simulink model "AWES3_CL_wTether_v4_PM"  (R2022a)
settings: Solver=ode3  StartTime=0  StopTime=simInit.TSIM  FixedStep=simInit.dt  RelTol=1e-3
values from neighbouring files (symbols this model uses):
  complex_tether_flag = 1    [run_sim.m]
  Ft_max = 1870    [run_sim.m]
  q = 0    [barrier_optimization.m]
  r = 0    [barrier_optimization.m]
  random_seed = [ 24335       17059       17670        1747]    [run_sim.m]
  safety_controller = false    [run_sim.m]
  turbulence = true    [run_sim.m]
undefined symbols (not defined in the file or in its folder): aeroModel, alpha_max, alpha_min, alpha_options, base_windspeed, constr, DiscIntNeverNeededParam, dx, ENVMT, F, grid_max, grid_min, HDBK, I_table, Light, MIL, mu_max, mu_min, mu_options, P_AP2, params, SampleTime, simInit, T, u0_sim, winchParameter, x0_sim
libraries: simulink x30, aerolibwind2 x14, dspstat3 x2, pid_lib x1, aerolibwindfilters x1, aerolibcommonsys x1, matrix_library x1
(part 3 of 5)

== system AWES3_CL_wTether_v4_PM/FlightController/Retraction/CalculateAttitudeCmds ==
  pathangles_k_cmd : Inport
  Ft_set : Inport  Port=2
  F_t_m : Inport  Port=3
  airdata : Inport  Port=4
  v_w_O : Inport  Port=5
  v_k_O : Inport  Port=6
  p_G_O : Inport  Port=7
  pathangles_a : Inport  Port=8
  mu_a : Inport  Port=9
  Demux{1..4} (4 alike) : Demux  Outputs=2
  Dot Product : DotProduct  OutDataTypeStr=Inherit: Inherit via internal rule
  FlightPathLoopRetraction : Subsystem
  FlightpathReferenceModels : Subsystem
  Gain : Gain  Gain=0.5*1.225
  Mux1 : Mux  Commented=on  Inputs=3
  Mux3 : Mux  Commented=on  Inputs=3
  PIController_opt : Subsystem
  Product : Product
  Saturation : Saturate  UpperLimit=constr.alpha_a_max  LowerLimit=constr.alpha_a_min
  Scope1 : Scope  Commented=on
  Scope2 : Scope  Commented=on
  Selector : Selector  InputPortWidth=3  IndexOptions=Index vector (dialog)  Indices=1  OutputSizes=1
  Selector1 : Selector  InputPortWidth=3  IndexOptions=Index vector (dialog)  Indices=3  OutputSizes=1
  Sqrt : Sqrt
  Sum : Sum  Inputs=|+-
  Sum1 : Sum  Inputs=|+-
  Terminator : Terminator
  Terminator1 : Terminator
  TrafoPathKin2PathAero : MATLAB Function  TreatAsAtomicUnit=on
  mu_a_cmd : Outport  VectorParamsAs1DForOutWhenUnconnected=off
  alpha_cmd : Outport  Port=2  VectorParamsAs1DForOutWhenUnconnected=off
  wires:
  FlightPathLoopRetraction/1(mu_a_c) -> mu_a_cmd/1
  pathangles_a/1 -> FlightPathLoopRetraction/5(pathangles_a), Demux4/1, PIController_opt/3(path_angles_a)
  p_G_O/1 -> FlightPathLoopRetraction/6(p_G_O)
  FlightPathLoopRetraction/3(Ft) -> Terminator1/1
  FlightPathLoopRetraction/4(push_mode) -> Terminator/1
  FlightPathLoopRetraction/6(gamma_dot_real) -> Sum1/2
  pathangles_k_cmd/1 -> Demux2/1
  Ft_set/1 -> FlightPathLoopRetraction/2(F_t_set)
  Selector1/1 -> TrafoPathKin2PathAero/6(beta)
  TrafoPathKin2PathAero/2(gamma_a) -> FlightpathReferenceModels/2(gamma_cmd), Mux3/1
  TrafoPathKin2PathAero/1(chi_a) -> FlightpathReferenceModels/1(chi_cmd), Mux1/1
  Selector/1 -> TrafoPathKin2PathAero/2(Va), Product/1, Product/2  "Va"
  Sqrt/1 -> TrafoPathKin2PathAero/1(Vg)
  Dot Product/1 -> Sqrt/1
  FlightPathLoopRetraction/2(alpha_a_c) -> Saturation/1
  PIController_opt/1(nu_a_path) -> Demux1/1, FlightPathLoopRetraction/3(nu_a_path)
  Sum1/1 -> FlightpathReferenceModels/4(gamma_hedge)
  FlightPathLoopRetraction/5(chi_dot_real) -> Sum/2
  Demux1/2 -> Sum1/1
  Demux1/1 -> Sum/1
  FlightpathReferenceModels/1(xD_ref) -> PIController_opt/1(dot_Ref)
  Demux2/1 -> TrafoPathKin2PathAero/4(chi_k)
  FlightpathReferenceModels/2(x_ref) -> Demux3/1, PIController_opt/2(x_ref)
  Demux2/2 -> TrafoPathKin2PathAero/3(gamma_k)
  Demux3/1 -> Mux1/2
  Demux4/2 -> Mux3/3
  Demux3/2 -> Mux3/2
  Demux4/1 -> Mux1/3
  Product/1 -> Gain/1
  Gain/1 -> FlightpathReferenceModels/5(dynamic_pressure)
  Mux1/1 -> Scope1/1
  Mux3/1 -> Scope2/1
  Sum/1 -> FlightpathReferenceModels/3(chi_hedge)
  F_t_m/1 -> FlightPathLoopRetraction/1(F_t_m)
  airdata/1 -> FlightPathLoopRetraction/4(airdata), Selector1/1, Selector/1
  v_w_O/1 -> TrafoPathKin2PathAero/5(v_w_O)
  v_k_O/1 -> Dot Product/2, Dot Product/1
  mu_a/1 -> FlightPathLoopRetraction/7(mu_a)
  Saturation/1 -> alpha_cmd/1

== system AWES3_CL_wTether_v4_PM/FlightController/Retraction/GuidanceFlatEarth ==
  pos_G_O : Inport
  "vel_K_O " : Inport  Port=2
  phi0_retraction : Inport  Port=3
  Va : Inport  Port=4
  Chart : Stateflow chart  TreatAsAtomicUnit=on  mask{vamin_max=params.vamin_max, vamin=params.vamin, vamax=params.vamax, vamax_min=params.vamax_min}
  Constant : Constant  Value=params.vamin_max
  Delay1 : Delay  DelayLength=1  InitialConditionSource=Input port  InitialCondition=zeros(3,1)
      settings: InputPortMap=u0,p4
  Delay2 : Delay  DelayLength=1
  Dot Product3 : DotProduct  OutDataTypeStr=Inherit: Inherit via internal rule
  Gain1 : Gain  Gain=params.KpVaControl
  Gain3 : Gain  Gain=-1
  Gain5 : Gain  Gain=-1
  MATLAB Function1 : MATLAB Function  TreatAsAtomicUnit=on
  Mux : Mux  Inputs=2
  Mux1 : Mux  Inputs=2
  Saturation1 : Saturate  UpperLimit=constr.gamma_retraction_max  LowerLimit=constr.gamma_retraction_min
  Sqrt1 : Sqrt
  Sum : Sum  Inputs=|+-
  Sum1 : Sum  Inputs=++|
  Switch : Switch  Criteria=u2 > Threshold  SaturateOnIntegerOverflow=off  InputSameDT=off
  Terminator1 : Terminator
  calculateTransitionTrigger1 : MATLAB Function  TreatAsAtomicUnit=on
  d2r : Gain  Gain=pi/180
  approachFlag : Outport  VectorParamsAs1DForOutWhenUnconnected=off
  course_path : Outport  Port=2  VectorParamsAs1DForOutWhenUnconnected=off
  transition_flag : Outport  Port=3  VectorParamsAs1DForOutWhenUnconnected=off
  flag_pos_W : Outport  Port=4  VectorParamsAs1DForOutWhenUnconnected=off
  retraction_path_error : Outport  Port=5  VectorParamsAs1DForOutWhenUnconnected=off
  target_W : Outport  Port=6  VectorParamsAs1DForOutWhenUnconnected=off
  wires:
  Mux/1 -> course_path/1
  calculateTransitionTrigger1/2(transition_flag) -> transition_flag/1
  calculateTransitionTrigger1/7(flag_pos_y_W) -> flag_pos_W/1
  pos_G_O/1 -> Gain3/1, calculateTransitionTrigger1/2(pos_G_O_m)
  Delay1/1 -> Gain5/1, Delay1/1
  "vel_K_O "/1 -> Dot Product3/1, Dot Product3/2, MATLAB Function1/1(vel_k_O)
  Gain3/1 -> Delay1/2
  Dot Product3/1 -> Sqrt1/1
  Sqrt1/1 -> calculateTransitionTrigger1/4(v_k_tot)
  Gain5/1 -> calculateTransitionTrigger1/1(pos_init_retraction_O)
  calculateTransitionTrigger1/3(chi_k_cmd) -> Mux/1
  MATLAB Function1/2(vel_k_h_W) -> calculateTransitionTrigger1/3(vk_xy)
  MATLAB Function1/1(vel_k_down_W) -> Terminator1/1
  Saturation1/1 -> Mux/2  "gamma"
  calculateTransitionTrigger1/4(d_horizontal) -> Mux1/1
  calculateTransitionTrigger1/5(d_vertical) -> Mux1/2
  phi0_retraction/1 -> calculateTransitionTrigger1/5(phi0_retraction)
  calculateTransitionTrigger1/8(approachFlag) -> Delay2/1  "approachFlag"
  Delay2/1 -> approachFlag/1
  Chart/1(speed_by_pitch) -> Switch/2
  Switch/1 -> Saturation1/1
  Sum/1 -> Gain1/1
  Constant/1 -> Sum/2
  Va/1 -> calculateTransitionTrigger1/6(Va), Sum/1, Chart/2(va)  "va"
  Sum1/1 -> Switch/1
  d2r/1 -> Sum1/2
  calculateTransitionTrigger1/6(gamma_k_cmd) -> Sum1/1, Switch/3
  Gain1/1 -> d2r/1
  calculateTransitionTrigger1/9(flare_flag) -> Chart/1(flare_flag)  "flare_flag"
  Mux1/1 -> retraction_path_error/1
  calculateTransitionTrigger1/1(target_W) -> target_W/1

== system AWES3_CL_wTether_v4_PM/FlightController/Traction/FlightPathLoopTraction ==
  Ft_set : Inport
  F_a_B_est : Inport  Port=2  PortDimensions=[3,1]
  nu_chi : Inport  Port=3
  nu_gamma : Inport  Port=4
  pos_G_O : Inport  Port=5  PortDimensions=[3,1]
  airdata : Inport  Port=6  PortDimensions=[3,1]
  pathangles_k : Inport  Port=7  PortDimensions=[2,1]
  pathangles_a : Inport  Port=8  PortDimensions=[2,1]
  v_k_B : Inport  Port=9  PortDimensions=[3,1]
  mu_a_cmd : Inport  Port=10
  Constant : Constant  Value=0
  Delay{,2..5} (5 alike) : Delay  DelayLength=1  ExternalReset=Falling
      settings: InputPortMap=u0,r5
  Delay1 : Delay  DelayLength=1  InitialConditionSource=Input port  ExternalReset=Falling
      settings: InputPortMap=u0,r5,p4
  Demux : Demux  Outputs=2
  Demux1 : Demux  Outputs=2
  Demux2 : Demux  Outputs=2
  EstimatePlantResponse : Subsystem
  MATLAB Function : MATLAB Function  TreatAsAtomicUnit=on
  Mux : Mux  Inputs=2
  Saturation : Saturate  UpperLimit=constr.alpha_a_max  LowerLimit=constr.alpha_a_min
  Sum{,1..3} (4 alike) : Sum  Inputs=|+-
  inversionPathDynamics : MATLAB Function  TreatAsAtomicUnit=on
  inversionPathDynamics1 : MATLAB Function  Commented=on  TreatAsAtomicUnit=on
  mu_a_c_traction : Outport  PortDimensions=1  VectorParamsAs1DForOutWhenUnconnected=off
  alpha_rq : Outport  Port=2  PortDimensions=1  VectorParamsAs1DForOutWhenUnconnected=off
  wires:
  F_a_B_est/1 -> inversionPathDynamics/4(F_a_B_est)
  Demux1/1 -> inversionPathDynamics/6(chi_k)
  pathangles_a/1 -> inversionPathDynamics/9(pathangles_a)
  inversionPathDynamics/1(mu_a) -> mu_a_c_traction/1
  Mux/1 -> Demux/1
  Demux/2 -> inversionPathDynamics/3(nu_gamma_k)
  Demux/1 -> inversionPathDynamics/2(nu_chi_k)
  inversionPathDynamics/2(mu_k_c) -> EstimatePlantResponse/1(mu_k_sat)
  inversionPathDynamics/3(alpha_rq) -> Saturation/1
  inversionPathDynamics/4(dphi) -> EstimatePlantResponse/2(dphi)
  Delay1/1 -> inversionPathDynamics/11(L_rq_old)
  Delay/1 -> inversionPathDynamics/12(mu_a_old)
  MATLAB Function/1(L_rq) -> Delay1/3
  inversionPathDynamics/5(L_rq) -> Delay1/1
  Demux1/2 -> inversionPathDynamics/7(gamma_k)
  airdata/1 -> EstimatePlantResponse/8(airdata), inversionPathDynamics/10(airdata), MATLAB Function/1(airdata)
  pathangles_k/1 -> EstimatePlantResponse/5(chi_gamma_k), Demux1/1
  v_k_B/1 -> EstimatePlantResponse/7(v_k_B), inversionPathDynamics/8(v_k_B)
  pos_G_O/1 -> inversionPathDynamics/5(pos_O), EstimatePlantResponse/6(pos_O)
  Ft_set/1 -> EstimatePlantResponse/3(Ft), inversionPathDynamics/1(Ft_set)
  Delay5/1 -> Sum3/1
  nu_chi/1 -> Sum/1
  Sum3/1 -> Sum/2
  Delay4/1 -> Sum2/2
  Delay3/1 -> Sum3/2
  Demux2/2 -> Delay4/1
  Sum1/1 -> Delay2/1, Mux/2
  Sum/1 -> Delay5/1, Mux/1
  Delay2/1 -> Sum2/1
  EstimatePlantResponse/1(pathAngleRate) -> Demux2/1
  nu_gamma/1 -> Sum1/1
  Demux2/1 -> Delay3/1
  Sum2/1 -> Sum1/2
  mu_a_cmd/1 -> Delay/1
  Constant/1 -> Delay/2, Delay1/2, Delay2/2, Delay5/2, Delay4/2, Delay3/2
  Saturation/1 -> EstimatePlantResponse/4(alpha_rq), alpha_rq/1

== system AWES3_CL_wTether_v4_PM/FlightController/Traction/Ft_set_smoothing ==
  F_t_m : Inport
  Data Type Conversion : DataTypeConversion  OutDataTypeStr=boolean  SaturateOnIntegerOverflow=off  RndMeth=Floor
  force switch1 : Subsystem  Commented=on
  force switch2 : Subsystem
  recommend_switch : Outport
  Ft_set_out : Outport  Port=2
  wires:
  F_t_m/1 -> force switch2/1(u), Ft_set_out/1
  force switch2/1(Out) -> Data Type Conversion/1
  Data Type Conversion/1 -> recommend_switch/1

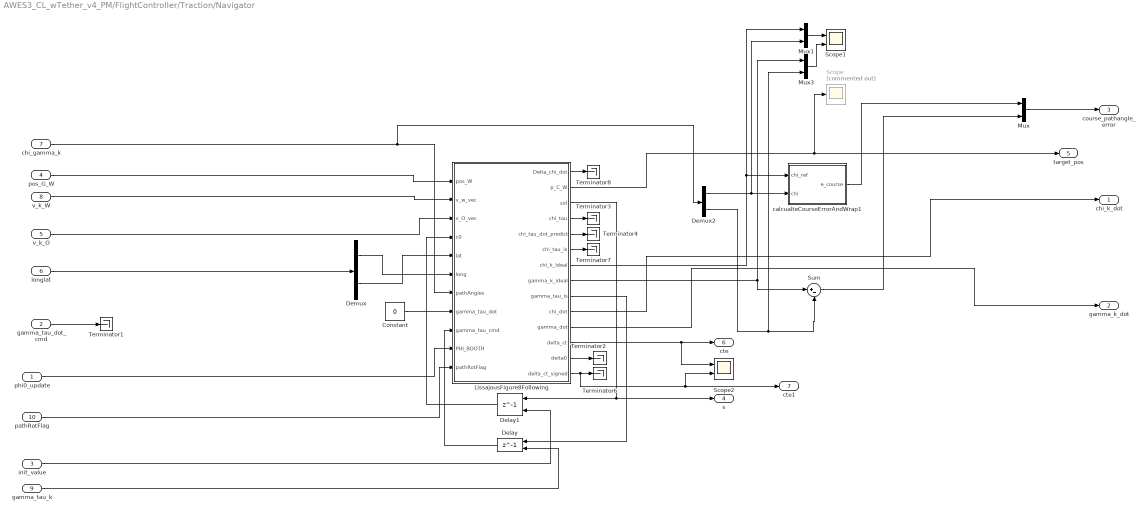
== system AWES3_CL_wTether_v4_PM/FlightController/Traction/Navigator ==
  phi0_update : Inport
  gamma_tau_dot_cmd : Inport  Port=2
  init_value : Inport  Port=3
  pos_G_W : Inport  Port=4
  v_k_O : Inport  Port=5
  longlat : Inport  Port=6  PortDimensions=2
  chi_gamma_k : Inport  Port=7
  v_k_W : Inport  Port=8
  gamma_tau_k : Inport  Port=9
  pathRotFlag : Inport  Port=10
  Constant : Constant  Value=0
  Delay : Delay  DelayLength=1  InitialConditionSource=Input port  InitialCondition=0
      settings: InputPortMap=u0,p4
  Delay1 : Delay  DelayLength=1  InitialConditionSource=Input port  InitialCondition=pi/2
      settings: InputPortMap=u0,p4
  Demux : Demux  Outputs=2
  Demux2 : Demux  Outputs=2
  LissajousFigure8Following : MATLAB Function  TreatAsAtomicUnit=on
  Mux : Mux  Inputs=2
  Mux1 : Mux  Inputs=2
  Mux3 : Mux  Inputs=2
  Scope : Scope  Commented=on
  Scope1 : Scope  NumInputPorts=2
  Scope2 : Scope  NumInputPorts=2
  Sum : Sum  Inputs=|+-
  Terminator{1..4,6..8} (7 alike) : Terminator
  calcualteCourseErrorAndWrap1 : MATLAB Function  TreatAsAtomicUnit=on
  chi_k_dot : Outport  PortDimensions=1  VectorParamsAs1DForOutWhenUnconnected=off
  gamma_k_dot : Outport  Port=2  PortDimensions=1  VectorParamsAs1DForOutWhenUnconnected=off
  "course_pathangle_error " : Outport  Port=3  VectorParamsAs1DForOutWhenUnconnected=off
  s : Outport  Port=4  PortDimensions=1  VectorParamsAs1DForOutWhenUnconnected=off
  target_pos : Outport  Port=5  VectorParamsAs1DForOutWhenUnconnected=off
  cte : Outport  Port=6  PortDimensions=1  VectorParamsAs1DForOutWhenUnconnected=off
  cte1 : Outport  Port=7  PortDimensions=1  VectorParamsAs1DForOutWhenUnconnected=off
  wires:
  Mux3/1 -> Scope1/2
  Mux1/1 -> Scope1/1
  LissajousFigure8Following/2(p_C_W) -> target_pos/1, Scope/1
  Delay1/1 -> LissajousFigure8Following/4(c0)
  LissajousFigure8Following/3(sol) -> Delay1/1, s/1
  v_k_O/1 -> LissajousFigure8Following/3(v_O_vec)
  Demux/1 -> LissajousFigure8Following/6(long)
  calcualteCourseErrorAndWrap1/1(e_course) -> Mux/1
  LissajousFigure8Following/7(chi_k_ideal) -> calcualteCourseErrorAndWrap1/1(chi_ref), Mux1/1
  Demux2/1 -> calcualteCourseErrorAndWrap1/2(chi), Mux1/2
  Demux2/2 -> Mux3/2, Sum/2
  Mux/1 -> "course_pathangle_error "/1
  LissajousFigure8Following/11(gamma_dot) -> gamma_k_dot/1
  LissajousFigure8Following/10(chi_dot) -> chi_k_dot/1
  Sum/1 -> Mux/2
  Demux/2 -> LissajousFigure8Following/5(lat)
  LissajousFigure8Following/9(gamma_tau_is) -> Delay/1
  pos_G_W/1 -> LissajousFigure8Following/1(pos_W)
  longlat/1 -> Demux/1
  chi_gamma_k/1 -> LissajousFigure8Following/7(pathAngles), Demux2/1
  gamma_tau_dot_cmd/1 -> Terminator1/1
  init_value/1 -> Delay1/2
  Constant/1 -> LissajousFigure8Following/8(gamma_tau_dot)
  v_k_W/1 -> LissajousFigure8Following/2(v_w_vec)
  LissajousFigure8Following/13(delta0) -> Terminator2/1
  LissajousFigure8Following/4(chi_tau) -> Terminator3/1
  LissajousFigure8Following/12(delta_ct) -> Scope2/1, cte/1
  LissajousFigure8Following/14(delta_ct_signed) -> Scope2/2, cte1/1, Terminator6/1
  LissajousFigure8Following/6(chi_tau_is) -> Terminator7/1
  LissajousFigure8Following/8(gamma_k_ideal) -> Mux3/1, Sum/1
  phi0_update/1 -> LissajousFigure8Following/10(PHI_BOOTH)
  LissajousFigure8Following/5(chi_tau_dot_predict) -> Terminator4/1
  gamma_tau_k/1 -> Delay/2
  pathRotFlag/1 -> LissajousFigure8Following/11(pathRotFlag)
  LissajousFigure8Following/1(Delta_chi_dot) -> Terminator8/1
  Delay/1 -> LissajousFigure8Following/9(gamma_tau_cmd)

== system AWES3_CL_wTether_v4_PM/FlightController/Traction/PI_controller_course ==
  In1 : Inport
  Demux : Demux  Outputs=2
  PI_controller_course_chi : Subsystem
  PI_controller_course_gamma : Subsystem
  chi_error : Outport
  gamma_error : Outport  Port=2
  wires:
  PI_controller_course_chi/1(u_PI_fb) -> chi_error/1  "chi_error"
  In1/1 -> Demux/1
  Demux/1 -> PI_controller_course_chi/1(e_chi)
  PI_controller_course_gamma/1(u_PI_fb) -> gamma_error/1  "gamma_error"
  Demux/2 -> PI_controller_course_gamma/1(e_gamma)

== system AWES3_CL_wTether_v4_PM/FlightController/Traction/Subsystem ==
  alpha_safety_cmd : Inport
  safety_switch : Inport  Port=2
  alpha_NDI_cmd : Inport  Port=3
  Gain4 : Gain
  Integrator3 : Integrator  ExternalReset=rising  InitialConditionSource=external
  Sum5 : Sum  Inputs=|+-
  Switch3 : Switch  Criteria=u2 > Threshold  SaturateOnIntegerOverflow=off  InputSameDT=off
  alpha_cmd : Outport
  wires:
  alpha_safety_cmd/1 -> Switch3/1, Sum5/1
  Gain4/1 -> Integrator3/1
  Sum5/1 -> Gain4/1
  safety_switch/1 -> Switch3/2, Integrator3/2
  Switch3/1 -> alpha_cmd/1  "alpha_cmd"
  Integrator3/1 -> Sum5/2  "alpha_safety_smooth"
  alpha_NDI_cmd/1 -> Integrator3/3, Switch3/3

== system AWES3_CL_wTether_v4_PM/FlightController/Traction/Subsystem1 ==
  mu_safety_cmd : Inport
  safety_switch : Inport  Port=2
  mu_NDI_cmd : Inport  Port=3
  Gain3 : Gain
  Integrator1 : Integrator  ExternalReset=rising  InitialConditionSource=external
  Sum3 : Sum  Inputs=|+-
  Switch2 : Switch  Criteria=u2 > Threshold  SaturateOnIntegerOverflow=off  InputSameDT=off
  mu_cmd : Outport
  wires:
  safety_switch/1 -> Switch2/2, Integrator1/2
  Switch2/1 -> mu_cmd/1  "mu_cmd"
  Gain3/1 -> Integrator1/1
  Sum3/1 -> Gain3/1
  mu_NDI_cmd/1 -> Integrator1/3, Switch2/3
  Integrator1/1 -> Sum3/2  "mu_safety_smooth"
  mu_safety_cmd/1 -> Switch2/1, Sum3/1

== system AWES3_CL_wTether_v4_PM/FlightController/Traction/Subsystem2 ==
  alpha_safety_cmd : Inport
  safety_switch : Inport  Port=2
  alpha_NDI_cmd : Inport  Port=3
  Gain4 : Gain  Gain=params.w0_mu_a_emulation
  Integrator3 : Integrator  ExternalReset=rising  InitialConditionSource=external
  Sum5 : Sum  Inputs=|+-
  Switch3 : Switch  Criteria=u2 > Threshold  SaturateOnIntegerOverflow=off  InputSameDT=off
  alpha_cmd : Outport
  wires:
  alpha_safety_cmd/1 -> Sum5/1
  Gain4/1 -> Integrator3/1
  Sum5/1 -> Gain4/1
  alpha_NDI_cmd/1 -> Integrator3/3, Switch3/3
  safety_switch/1 -> Switch3/2, Integrator3/2
  Switch3/1 -> alpha_cmd/1  "alpha_cmd"
  Integrator3/1 -> Sum5/2, Switch3/1  "alpha_safety_smooth"

== system AWES3_CL_wTether_v4_PM/FlightController/Traction/Subsystem3 ==
  s : Inport
  sigma : Inport  Port=2
  recommend_switch : Inport  Port=3
  h_tau : Inport  Port=4
  Va : Inport  Port=5
  chi_a : Inport  Port=6
  gamma_a : Inport  Port=7
  tether_diff : Inport  Port=8
  Enable : EnablePort  StatesWhenEnabling=reset
  Max : MinMax  Inputs=2
  Safety control : MATLAB Function  TreatAsAtomicUnit=on
  Saturation : Saturate  UpperLimit=constr.alpha_a_max  LowerLimit=constr.alpha_a_min
  safety_switch : Outport
  mu_safety_cmd : Outport  Port=2
  alpha_safety_cmd : Outport  Port=3
  in_BRS : Outport  Port=4
  wires:
  Safety control/2(mu_a) -> mu_safety_cmd/1  "mu_safety_cmd"
  sigma/1 -> Safety control/2(sigma)
  h_tau/1 -> Safety control/3(h_tau)
  Max/1 -> safety_switch/1  "safety_switch"
  Va/1 -> Safety control/4(Va)
  gamma_a/1 -> Safety control/6(gamma_a)
  tether_diff/1 -> Safety control/7(tether_diff)
  s/1 -> Safety control/1(s)
  chi_a/1 -> Safety control/5(chi_a)
  Safety control/3(alpha_a) -> Saturation/1  "alpha_safety_cmd"
  Safety control/1(value) -> in_BRS/1, Max/1  "in_BRS"
  recommend_switch/1 -> Max/2
  Saturation/1 -> alpha_safety_cmd/1

== system AWES3_CL_wTether_v4_PM/FlightController/Traction/alpha_actuator_delay1 ==
  alpha_cmd : Inport
  Gain : Gain  Gain=params.w0_alpha_a_emulation
  Integrator : Integrator  InitialConditionSource=external
  Sum2 : Sum  Inputs=|+-
  alpha_is : Outport
  wires:
  Integrator/1 -> Sum2/2, alpha_is/1
  Gain/1 -> Integrator/1
  alpha_cmd/1 -> Integrator/2, Sum2/1
  Sum2/1 -> Gain/1

== system AWES3_CL_wTether_v4_PM/FlightController/Traction/mu_actuator_delay ==
  mu_cmd : Inport
  Gain : Gain  Gain=params.w0_mu_a_emulation
  Integrator : Integrator  InitialConditionSource=external
  Sum2 : Sum  Inputs=|+-
  mu_is : Outport
  wires:
  Integrator/1 -> Sum2/2, mu_is/1  "mu_is"
  Gain/1 -> Integrator/1
  mu_cmd/1 -> Integrator/2, Sum2/1
  Sum2/1 -> Gain/1

== system AWES3_CL_wTether_v4_PM/Aircraft_Winch_Tether/Subsystem/6DoFKinematics1/LowPassFilter ==
  In1 : Inport
  Gain : Gain  Gain=w0
  Integrator : Integrator  InitialCondition=x0
  Sum2 : Sum  Inputs=|+-
  Out1 : Outport  VectorParamsAs1DForOutWhenUnconnected=off
  wires:
  Gain/1 -> Integrator/1
  Sum2/1 -> Gain/1
  In1/1 -> Sum2/1
  Integrator/1 -> Out1/1, Sum2/2

== system AWES3_CL_wTether_v4_PM/Aircraft_Winch_Tether/WinchDynamicsAndControl /PureTorqueControl/PI-ForceController ==
  preSat : Inport
  retraction : Inport  Port=2
  controlDeficitDue2Sat : Inport  Port=3
  e_Ft : Inport  Port=4
  Constant : Constant  Value=base_windspeed
  Constant1 : Constant  Value=9
  Constant3 : Constant  Value=7
  Constant4 : Constant
  Discrete-Time Integrator1 : DiscreteIntegrator  ExternalReset=either  SampleTime=-1  UpperSaturationLimit=winchParameter.omega_max  LowerSaturationLimit=winchParameter.omega_min  ICPrevOutput=DiscIntNeverNeededParam  ICPrevScaledInput=DiscIntNeverNeededParam
  Divide : Product  Inputs=*/
  Gain1 : Gain  Gain=2
  Gain2 : Gain  Gain=2
  Gain3 : Gain  Gain=60
  Gain8 : Gain  Gain=params.ki_winch
  Gain9 : Gain  Gain=params.kp_winch
  HighWindGain1 : Gain  Gain=0.5
  LowWindGain1 : Gain  Gain=0.5
  Product1 : Product
  Saturation Dynamic : simulink/Discontinuities/Saturation Dynamic  OutMin=[]  OutMax=[]  OutDataTypeStr=Inherit: Same as second input  OutDataType=fixdt(1, 16)  OutScaling=2^-10  DoSatur=off
  Sum : Sum  Inputs=|+-
  Sum1 : Sum  Inputs=|+-
  Sum2 : Sum  Inputs=|++
  Sum3 : Sum  Inputs=|-+
  Sum8 : Sum
  clamping_logic : Subsystem
  TorqueCmd : Outport  VectorParamsAs1DForOutWhenUnconnected=off
  wires:
  Gain9/1 -> Gain2/1
  Gain8/1 -> Gain1/1
  clamping_logic/1(pre_integration_processed) -> Discrete-Time Integrator1/1
  Gain1/1 -> clamping_logic/2(preInt)
  Discrete-Time Integrator1/1 -> Sum8/1
  Sum8/1 -> TorqueCmd/1
  e_Ft/1 -> Gain9/1, Gain8/1
  retraction/1 -> Discrete-Time Integrator1/2
  Constant/1 -> Saturation Dynamic/2
  Constant3/1 -> Sum1/2, Sum/2, Saturation Dynamic/3
  Saturation Dynamic/1 -> Sum/1
  Divide/1 -> HighWindGain1/1, Sum3/1
  HighWindGain1/1 -> Sum2/1
  Constant4/1 -> Sum3/2
  Sum3/1 -> LowWindGain1/1
  LowWindGain1/1 -> Sum2/2
  Product1/1 -> Sum8/2
  Sum2/1 -> Product1/2
  Constant1/1 -> Saturation Dynamic/1, Sum1/1
  Sum/1 -> Divide/1
  Sum1/1 -> Divide/2
  controlDeficitDue2Sat/1 -> clamping_logic/3(control_def)
  preSat/1 -> clamping_logic/1(preSat)
  Gain2/1 -> Product1/1

== system AWES3_CL_wTether_v4_PM/Aircraft_Winch_Tether/WinchDynamicsAndControl /PureTorqueControl/Subsystem ==
  In1 : Inport
  Gain1 : Gain  Gain=params.winch_control_filter_w0*0.25
  Integrator : Integrator
  Sum1 : Sum  Inputs=|+-
  Out1 : Outport  VectorParamsAs1DForOutWhenUnconnected=off
  wires:
  Sum1/1 -> Gain1/1
  Integrator/1 -> Out1/1, Sum1/2  "F_t_m"
  Gain1/1 -> Integrator/1
  In1/1 -> Sum1/1

== system AWES3_CL_wTether_v4_PM/Aircraft_Winch_Tether/WinchDynamicsAndControl /PureTorqueControl1/PI-ForceController ==
  RetractionFlag : Inport
  controlDeficitDue2Sat : Inport  Port=2
  e_Ft : Inport  Port=3
  Abs : Abs  SaturateOnIntegerOverflow=off
  Compare To Constant : simulink/Logic and Bit Operations/Compare To Constant  relop=>=  const=1e-3  OutDataTypeStr=boolean
  Constant2 : Constant  Value=0
  Discrete-Time Integrator1 : DiscreteIntegrator  ExternalReset=rising  SampleTime=simInit.dt  UpperSaturationLimit=winchParameter.omega_max  LowerSaturationLimit=winchParameter.omega_min  ICPrevOutput=DiscIntNeverNeededParam  ICPrevScaledInput=DiscIntNeverNeededParam
  Gain11 : Gain  Gain=0.5
  Gain7 : Gain  Gain=0.14
  Gain8 : Gain  Gain=params.ki_winch
  Gain9 : Gain  Gain=params.kp_winch
  Logical Operator : Logic  Operator=OR  AllPortsSameDT=off  OutDataTypeStr=boolean
  Scope : Scope
  Sum8 : Sum
  Switch : Switch  Criteria=u2 > Threshold  SaturateOnIntegerOverflow=off  InputSameDT=off
  TorqueCmd : Outport  VectorParamsAs1DForOutWhenUnconnected=off
  wires:
  ? -> Discrete-Time Integrator1/2
  RetractionFlag/1 -> Logical Operator/1
  e_Ft/1 -> Gain8/1, Gain9/1
  controlDeficitDue2Sat/1 -> Abs/1
  Sum8/1 -> TorqueCmd/1
  Abs/1 -> Compare To Constant/1
  Discrete-Time Integrator1/1 -> Sum8/1, Scope/1
  Compare To Constant/1 -> Logical Operator/2
  Gain11/1 -> Switch/3
  Switch/1 -> Discrete-Time Integrator1/1
  Gain8/1 -> Gain11/1
  Logical Operator/1 -> Switch/2
  Gain7/1 -> Sum8/2
  Gain9/1 -> Gain7/1
  Constant2/1 -> Switch/1

== system AWES3_CL_wTether_v4_PM/Aircraft_Winch_Tether/WinchDynamicsAndControl /PureTorqueControl2/PI-ForceController ==
  retraction : Inport
  controlDeficitDue2Sat : Inport  Port=2
  e_Ft : Inport  Port=3
  Abs : Abs  SaturateOnIntegerOverflow=off
  Compare To Constant : simulink/Logic and Bit Operations/Compare To Constant  relop=>  const=0  OutDataTypeStr=boolean
  Compare To Constant1 : simulink/Logic and Bit Operations/Compare To Constant  relop=<  const=0  OutDataTypeStr=boolean
  Constant : Constant  Value=base_windspeed
  Constant1 : Constant  Value=9
  Constant2 : Constant  Value=0
  Constant3 : Constant  Value=7
  Constant4 : Constant
  Discrete-Time Integrator1 : DiscreteIntegrator  ExternalReset=either  SampleTime=-1  UpperSaturationLimit=winchParameter.omega_max  LowerSaturationLimit=winchParameter.omega_min  ICPrevOutput=DiscIntNeverNeededParam  ICPrevScaledInput=DiscIntNeverNeededParam
  Divide : Product  Inputs=*/
  Gain1 : Gain  Gain=0.5
  Gain8 : Gain  Gain=params.ki_winch
  Gain9 : Gain  Gain=params.kp_winch
  HighWindGain : Gain  Gain=0.5
  Logical Operator : Logic  AllPortsSameDT=off  OutDataTypeStr=boolean
  LowWindGain : Gain  Gain=0.4
  PID Controller : pid_lib/PID Controller  Controller=PID  Form=Parallel  TimeDomain=Continuous-time  UseExternalTs=off  SampleTime=-1  IntegratorMethod=Forward Euler  FilterMethod=Forward Euler  ControllerParametersSource=internal  P=1  I=1  D=0  UseFilter=on  N=100  TunerSelectOption=Transfer Function Based (PID Tuner App)  InitialConditionSource=internal  InitialConditionForIntegrator=0  InitialConditionForFilter=0  DifferentiatorICPrevScaledInput=0  ExternalReset=none  TrackingMode=off  Kt=1  LimitOutput=on  SatLimitsSource=internal  UpperSaturationLimit=inf  LowerSaturationLimit=-inf  LinearizeAsGain=on  AntiWindupMode=clamping  Kb=1  POutMin=[]  POutMax=[]  IOutMin=[]  IOutMax=[]  DOutMin=[]  DOutMax=[]  NOutMin=[]  NOutMax=[]  SumOutMin=[]  SumOutMax=[]  SaturationOutMin=[]  SaturationOutMax=[]  PParamMin=[]  PParamMax=[]  IParamMin=[]  IParamMax=[]  DParamMin=[]  DParamMax=[]  NParamMin=[]  NParamMax=[]  KbParamMin=[]  KbParamMax=[]  KtParamMin=[]  KtParamMax=[]  KbOutMin=[]  KbOutMax=[]  KtOutMin=[]  KtOutMax=[]  IntegratorOutMin=[]  IntegratorOutMax=[]  FilterOutMin=[]  FilterOutMax=[]  SumI1OutMin=[]  SumI1OutMax=[]  SumI2OutMin=[]  SumI2OutMax=[]  SumI3OutMin=[]  SumI3OutMax=[]  SumI4OutMin=[]  SumI4OutMax=[]  SumDOutMin=[]  SumDOutMax=[]  DifferentiatorOutMin=[]  DifferentiatorOutMax=[]  FilterDiffOutCoefMin=[]  FilterDiffOutCoefMax=[]  ReciprocalOutMin=[]  ReciprocalOutMax=[]  SumDenOutMin=[]  SumDenOutMax=[]  SumNumOutMin=[]  SumNumOutMax=[]  DivideOutMin=[]  DivideOutMax=[]  UdiffTsProdOutMin=[]  UdiffTsProdOutMax=[]  NTsProdOutMin=[]  NTsProdOutMax=[]  UintegralTsProdOutMin=[]  UintegralTsProdOutMax=[]  UngainTsProdOutMin=[]  UngainTsProdOutMax=[]  IntegratorContinuousStateAttributes=''  IntegratorStateMustResolveToSignalObject=off  IntegratorRTWStateStorageClass=Auto  FilterContinuousStateAttributes=''  FilterStateMustResolveToSignalObject=off  FilterRTWStateStorageClass=Auto  ParallelPVariant=InternalParameters  IdealPVariant=Disabled  IVariant=InternalParameters  DVariant=InternalParameters  IntegratorVariant=Continuous  SatVariant=Enabled  AWVariant=ContClampingParallel  PCopyVariant=Disabled  TRVariant=Disabled  FdbkBlocksVariant=Forward  IdealPFdbkVariant=Disabled  SatFdbkVariant=Disabled  DerivativeFilterVariant=ContFilter  NVariant=InternalParameters  NCopyVariant=Disabled  FilterICVariant=InternalICsFilter  IntegratorICVariant=InternalICs  ExternalResetVariant=Disabled  TRSumVariant=Passthrough  SumFdbkVariant=Disabled  SumVariant=Sum_PID  TsampFilterVariant=InternalTs  TsampNgainVariant=Passthrough  TsampIntegralVariant=Passthrough  ExternalSaturationOutDataTypeStr=Inherit: Same as second input
  Product : Product
  Product1 : Product
  Saturation Dynamic : simulink/Discontinuities/Saturation Dynamic  OutMin=[]  OutMax=[]  OutDataTypeStr=Inherit: Same as second input  OutDataType=fixdt(1, 16)  OutScaling=2^-10  DoSatur=off
  Scope : Scope
  Sign : Signum
  Sign1 : Signum
  Sum : Sum  Inputs=|+-
  Sum1 : Sum  Inputs=|+-
  Sum2 : Sum  Inputs=|++
  Sum3 : Sum  Inputs=|-+
  Sum8 : Sum
  Switch : Switch  Criteria=u2 > Threshold  SaturateOnIntegerOverflow=off  InputSameDT=off
  TorqueCmd : Outport  VectorParamsAs1DForOutWhenUnconnected=off
  wires:
  Sum1/1 -> Divide/2
  Sum/1 -> Divide/1
  Constant1/1 -> Sum1/1, Saturation Dynamic/1
  Sum2/1 -> Product1/2
  Product1/1 -> Sum8/2
  LowWindGain/1 -> Sum2/2
  Sum3/1 -> LowWindGain/1
  Constant4/1 -> Sum3/2
  HighWindGain/1 -> Sum2/1
  Divide/1 -> HighWindGain/1, Sum3/1
  Saturation Dynamic/1 -> Sum/1
  Constant3/1 -> Saturation Dynamic/3, Sum/2, Sum1/2
  Constant/1 -> Saturation Dynamic/2
  retraction/1 -> Discrete-Time Integrator1/2
  Logical Operator/1 -> Switch/2
  Compare To Constant1/1 -> Logical Operator/1
  Product/1 -> Compare To Constant1/1
  Sign/1 -> Product/2
  Sign1/1 -> Product/1
  e_Ft/1 -> Gain8/1, Gain9/1, Sign1/1
  controlDeficitDue2Sat/1 -> Abs/1, Sign/1
  Sum8/1 -> TorqueCmd/1
  Abs/1 -> Compare To Constant/1
  Discrete-Time Integrator1/1 -> Sum8/1, Scope/1
  Compare To Constant/1 -> Logical Operator/2
  Gain1/1 -> Switch/3
  Switch/1 -> Discrete-Time Integrator1/1
  Gain8/1 -> Gain1/1
  Gain9/1 -> Product1/1
  Constant2/1 -> Switch/1

== system AWES3_CL_wTether_v4_PM/Aircraft_Winch_Tether/WindfieldModel/Subsystem1/Subsystem ==
  Altitude : Inport  Unit=m
  Airspeed : Inport  Port=2  Unit=m/s
  DCM : Inport  Port=3  Unit=1  PortDimensions=[3 3]
  (u,v,w) : Selector  InputPortWidth=4  IndexOptions=Index vector (dialog)  Indices=[1 2 3]  OutputSizes=1
  Angle Conversion : aerolibwind2/Dryden Wind Turbulence Model  (Continuous (+q -r))/Angle Conversion  SystemSampleTime=-1  VariantActivationTime=update diagram  Latency=0  AutoFrameSizeCalculation=off
      settings: SourceProductBaseCode=AE
  Bus Creator : BusCreator  Inputs=3
  Disallow CGS : UnitConfiguration  UnitSystemsStr=English,SI,SI (extended)  AllowAllUnitSystems=off
  Filters on angular rates : aerolibwind2/Dryden Wind Turbulence Model  (Continuous (+q -r))/Filters on angular rates  SystemSampleTime=-1  VariantActivationTime=update diagram  Latency=0  AutoFrameSizeCalculation=off
      settings: SourceProductBaseCode=AE
  Filters on velocities : aerolibwindfilters/Dryden Continuous Filters  SystemSampleTime=-1  VariantActivationTime=update diagram  Latency=0  AutoFrameSizeCalculation=off
      settings: SourceProductBaseCode=AE
  Length Conversion : aerolibwind2/Dryden Wind Turbulence Model  (Continuous (+q -r))/Length Conversion  SystemSampleTime=-1  VariantActivationTime=update diagram  Latency=0  AutoFrameSizeCalculation=off
      settings: SourceProductBaseCode=AE
  Length Conversion1 : aerolibwind2/Dryden Wind Turbulence Model  (Continuous (+q -r))/Length Conversion1  SystemSampleTime=-1  VariantActivationTime=update diagram  Latency=0  AutoFrameSizeCalculation=off
      settings: SourceProductBaseCode=AE
  Mux : Mux  Inputs=3
  Mux1 : Mux  Inputs=3
  RMS turbulence intensities : aerolibwind2/Dryden Wind Turbulence Model  (Continuous (+q -r))/RMS turbulence  intensities  SystemSampleTime=-1  VariantActivationTime=update diagram  Latency=0  AutoFrameSizeCalculation=off
      settings: SourceProductBaseCode=AE
  Select angular rates : aerolibwind2/Dryden Wind Turbulence Model  (Continuous (+q -r))/Select angular rates  SystemSampleTime=-1  VariantActivationTime=update diagram  Latency=0  AutoFrameSizeCalculation=off
      settings: SourceProductBaseCode=AE
  Select velocities : aerolibwind2/Dryden Wind Turbulence Model  (Continuous (+q -r))/Select velocities  SystemSampleTime=-1  VariantActivationTime=update diagram  Latency=0  AutoFrameSizeCalculation=off
      settings: SourceProductBaseCode=AE
  Turbulence scale lengths : aerolibwind2/Dryden Wind Turbulence Model  (Continuous (+q -r))/Turbulence scale lengths  SystemSampleTime=-1  VariantActivationTime=update diagram  Latency=0  AutoFrameSizeCalculation=off
      settings: SourceProductBaseCode=AE
  Unit Conversion : UnitConversion
  Velocity Conversion : aerolibwind2/Dryden Wind Turbulence Model  (Continuous (+q -r))/Velocity Conversion  SystemSampleTime=-1  VariantActivationTime=update diagram  Latency=0  AutoFrameSizeCalculation=off
      settings: SourceProductBaseCode=AE
  Velocity Conversion2 : aerolibwind2/Dryden Wind Turbulence Model  (Continuous (+q -r))/Velocity Conversion2  SystemSampleTime=-1  VariantActivationTime=update diagram  Latency=0  AutoFrameSizeCalculation=off
      settings: SourceProductBaseCode=AE
  White Noise : aerolibcommonsys/Tunable White Noise  pwr=[1 1 1 1]*pi  Ts=0.1  seed=random_seed
      settings: SourceProductBaseCode=AE
  Wind direction : Constant  Value=Wdeg  OutDataTypeStr=Inherit: Inherit via back propagation
  Windspeed at 20ft (6m) : Constant  Value=W20  OutDataTypeStr=Inherit: Inherit via back propagation
  Wingspan : Constant  Value=Wingspan  OutDataTypeStr=Inherit: Inherit via back propagation
  p : Selector  InputPortWidth=4  IndexOptions=Index vector (dialog)  Indices=[4]  OutputSizes=1
  ug,vg,wg : Outport  Unit=m/s  VectorParamsAs1DForOutWhenUnconnected=off
  pg,qg,rg : Outport  Port=2  VectorParamsAs1DForOutWhenUnconnected=off
  wires:
  Select angular rates/2 -> Mux1/2
  Wingspan/1 -> Length Conversion1/1
  Select angular rates/1 -> Mux1/1
  Turbulence scale lengths/1 -> Filters on velocities/2
  Filters on angular rates/2 -> Select angular rates/2  "qgw"
  Mux1/1 -> pg,qg,rg/1
  Bus Creator/1 -> Select velocities/1, Select angular rates/4
  Filters on velocities/1 -> Select velocities/2  "ugw"
  Wind direction/1 -> Angle Conversion/1
  Windspeed at 20ft (6m)/1 -> Velocity Conversion2/1
  Filters on velocities/2 -> Select velocities/3, Filters on angular rates/1  "vgw"
  Altitude/1 -> Length Conversion/1
  Turbulence scale lengths/3 -> Filters on velocities/4, Filters on angular rates/4
  Velocity Conversion2/1 -> RMS turbulence intensities/2
  Airspeed/1 -> Velocity Conversion/1
  Filters on velocities/3 -> Select velocities/4, Filters on angular rates/2  "wgw"
  White Noise/1 -> p/1, (u,v,w)/1
  (u,v,w)/1 -> Filters on velocities/1
  RMS turbulence intensities/2 -> Filters on velocities/6
  Unit Conversion/1 -> ug,vg,wg/1
  Filters on angular rates/3 -> Select angular rates/3  "rgw"
  Angle Conversion/1 -> Bus Creator/2  "Wdeg"
  DCM/1 -> Bus Creator/1  "DCM"
  RMS turbulence intensities/1 -> Filters on velocities/5
  Velocity Conversion/1 -> Filters on velocities/8, Filters on angular rates/3
  Length Conversion1/1 -> Filters on angular rates/7
  Filters on angular rates/1 -> Select angular rates/1  "pgw"
  Select angular rates/3 -> Mux1/3
  p/1 -> Filters on angular rates/6
  Turbulence scale lengths/2 -> Filters on velocities/3
  Mux/1 -> Unit Conversion/1
  RMS turbulence intensities/3 -> Filters on velocities/7, Filters on angular rates/5
  Length Conversion/1 -> Turbulence scale lengths/1, RMS turbulence intensities/1, Bus Creator/3  "altitude"
  Select velocities/1 -> Mux/1  "ugw"
  Select velocities/3 -> Mux/3  "wgw"
  Select velocities/2 -> Mux/2  "vgw"

== system AWES3_CL_wTether_v4_PM/FlightController/Retraction/CalculateAttitudeCmds/FlightPathLoopRetraction ==
  F_t_m : Inport
  F_t_set : Inport  Port=2
  nu_a_path : Inport  Port=3
  airdata : Inport  Port=4
  pathangles_a : Inport  Port=5
  p_G_O : Inport  Port=6
  mu_a : Inport  Port=7
  Constant : Constant  Value=0
  Constant1 : Constant  Value=6
  Delay : Delay  DelayLength=1  InitialConditionSource=Input port
      settings: InputPortMap=u0,p4
  Delay1 : Delay  DelayLength=1  InitialConditionSource=Input port
      settings: InputPortMap=u0,p4
  Demux : Demux  Outputs=2
  MATLAB Function : MATLAB Function  TreatAsAtomicUnit=on
  Selector : Selector  InputPortWidth=2  IndexOptions=Index vector (dialog)  Indices=2  OutputSizes=1
  Selector1 : Selector  InputPortWidth=2  IndexOptions=Index vector (dialog)  Indices=1  OutputSizes=1
  Terminator : Terminator
  inversionPathDynamics : MATLAB Function  TreatAsAtomicUnit=on
  mu_a_c : Outport  PortDimensions=1  VectorParamsAs1DForOutWhenUnconnected=off
  alpha_a_c : Outport  Port=2  PortDimensions=1  VectorParamsAs1DForOutWhenUnconnected=off
  Ft : Outport  Port=3  VectorParamsAs1DForOutWhenUnconnected=off
  push_mode : Outport  Port=4  PortDimensions=1  VectorParamsAs1DForOutWhenUnconnected=off
  chi_dot_real : Outport  Port=5  PortDimensions=1  VectorParamsAs1DForOutWhenUnconnected=off
  gamma_dot_real : Outport  Port=6  PortDimensions=1  VectorParamsAs1DForOutWhenUnconnected=off
  wires:
  p_G_O/1 -> inversionPathDynamics/5(pos_O)
  Selector/1 -> inversionPathDynamics/7(gamma_a)
  pathangles_a/1 -> Selector/1, Selector1/1
  airdata/1 -> inversionPathDynamics/8(airdata), MATLAB Function/1(airdata)
  MATLAB Function/1(L_rq) -> Delay/2
  inversionPathDynamics/1(mu_a_c) -> Delay1/1, mu_a_c/1
  Delay1/1 -> inversionPathDynamics/12(mu_a_c_old)
  Delay/1 -> inversionPathDynamics/10(Lrq_old)
  Constant1/1 -> inversionPathDynamics/1(flightMode)
  nu_a_path/1 -> Demux/1
  Demux/2 -> inversionPathDynamics/3(nu_gamma_a)
  Demux/1 -> inversionPathDynamics/2(nu_chi_a)
  inversionPathDynamics/2(alpha_a_c) -> alpha_a_c/1
  Selector1/1 -> inversionPathDynamics/6(chi_a)
  Constant/1 -> inversionPathDynamics/9(ddt_v_w_x_O)
  mu_a/1 -> inversionPathDynamics/11(mu_a), Delay1/2
  inversionPathDynamics/3(L_rq) -> Delay/1
  inversionPathDynamics/4(push_mode) -> push_mode/1
  inversionPathDynamics/5(chi_dot_real) -> chi_dot_real/1
  inversionPathDynamics/6(gamma_dot_real) -> gamma_dot_real/1
  F_t_set/1 -> inversionPathDynamics/4(f_t), Ft/1
  F_t_m/1 -> Terminator/1

== system AWES3_CL_wTether_v4_PM/FlightController/Retraction/CalculateAttitudeCmds/FlightpathReferenceModels ==
  chi_cmd : Inport
  gamma_cmd : Inport  Port=2
  chi_hedge : Inport  Port=3
  gamma_hedge : Inport  Port=4
  dynamic_pressure : Inport  Port=5
  Mux2 : Mux  Inputs=2
  Mux3 : Mux  Inputs=2
  SecondOrderReferenceModel_Path2 : Subsystem  Commented=on  mask{omega0=params.w0_gamma_retraction, zeta0=1, y_max=80*pi/180, y_min=-80*pi/180, yd_max=inf, yd_min=-inf, y2d_max=inf, y2d_min=-inf}
  SecondOrderReferenceModel_course : Subsystem  mask{omega0_max=params.w0_chi_retraction_max, omega0_min=params.w0_chi_retraction_min, dynP_max=1.5312e+03, dynP_min=245.0000, zeta0=1, y_max=inf, y_min=-inf, yd_max=inf, yd_min=-inf, y2d_max=inf, y2d_min=-inf}
  SecondOrderReferenceModel_mu_a : Subsystem  Commented=on  mask{omega0_max=params.w0_mu_traction*1.2, omega0_min=params.w0_mu_traction*0.8, dynP_max=1.5312e+03, dynP_min=245.0000, zeta0=1, y_max=inf, y_min=-inf, yd_max=inf, yd_min=-inf, y2d_max=inf, y2d_min=-inf}
      mask prompts: dynP_max "max. dynamic pressure"; dynP_min "min. dynamic pressure"
  SecondOrderReferenceModel_pathangle : Subsystem  mask{omega0_max=params.w0_gamma_retraction_max, omega0_min=params.w0_gamma_retraction_min, dynP_max=1.5312e+03, dynP_min=245.0000, zeta0=1, y_max=inf, y_min=-inf, yd_max=inf, yd_min=-inf, y2d_max=inf, y2d_min=-inf}
  xD_ref : Outport  VectorParamsAs1DForOutWhenUnconnected=off
  x_ref : Outport  Port=2  VectorParamsAs1DForOutWhenUnconnected=off
  wires:
  dynamic_pressure/1 -> SecondOrderReferenceModel_course/3(dynamic_pressure), SecondOrderReferenceModel_pathangle/3(dynamic_pressure)
  gamma_hedge/1 -> SecondOrderReferenceModel_pathangle/2(hedge)
  chi_hedge/1 -> SecondOrderReferenceModel_course/2(hedge)
  gamma_cmd/1 -> SecondOrderReferenceModel_pathangle/1(y_cmd)
  chi_cmd/1 -> SecondOrderReferenceModel_course/1(y_cmd)
  Mux3/1 -> xD_ref/1
  Mux2/1 -> x_ref/1
  SecondOrderReferenceModel_course/1(y_ref) -> Mux2/1
  SecondOrderReferenceModel_pathangle/1(y_ref) -> Mux2/2
  SecondOrderReferenceModel_course/2(y_ref_dot) -> Mux3/1
  SecondOrderReferenceModel_pathangle/2(y_ref_dot) -> Mux3/2

== system AWES3_CL_wTether_v4_PM/FlightController/Retraction/CalculateAttitudeCmds/PIController_opt ==
  dot_Ref : Inport
  x_ref : Inport  Port=2
  path_angles_a : Inport  Port=3
  CircleP1 : Gain  Gain=params.Kp_gamma_retraction*1.2  Multiplication=Matrix(K*u)
  Demux : Demux  Outputs=2
  Demux1 : Demux  Outputs=2
  Discrete-Time Integrator : DiscreteIntegrator  SampleTime=-1  ICPrevOutput=DiscIntNeverNeededParam  ICPrevScaledInput=DiscIntNeverNeededParam
  Discrete-Time Integrator1 : DiscreteIntegrator  SampleTime=-1  ICPrevOutput=DiscIntNeverNeededParam  ICPrevScaledInput=DiscIntNeverNeededParam
  Gain : Gain
  Gain4 : Gain  Gain=params.Ki_chi_retraction*6  Multiplication=Matrix(K*u) (u vector)
  Gain5 : Gain  Gain=params.Ki_gamma_retraction*0.5  Multiplication=Matrix(K*u) (u vector)
  Kp : Gain  Gain=params.Kp_chi_retraction/4  Multiplication=Matrix(K*u)
  Mux : Mux  Inputs=2
  Mux1 : Mux  Inputs=2
  Selector2 : Selector  InputPortWidth=2  IndexOptions=Index vector (dialog)  Indices=1  OutputSizes=1
  Selector3 : Selector  InputPortWidth=2  IndexOptions=Index vector (dialog)  Indices=1  OutputSizes=1
  Selector4 : Selector  InputPortWidth=2  IndexOptions=Index vector (dialog)  Indices=2  OutputSizes=1
  Selector5 : Selector  InputPortWidth=2  IndexOptions=Index vector (dialog)  Indices=2  OutputSizes=1
  Sum : Sum  Inputs=|+-
  Sum{1..4} (4 alike) : Sum  Inputs=|++
  wrapCourse : MATLAB Function  TreatAsAtomicUnit=on
  nu_a_path : Outport  VectorParamsAs1DForOutWhenUnconnected=off
  wires:
  Mux1/1 -> Demux1/1
  Mux/1 -> nu_a_path/1  "nu_R"
  dot_Ref/1 -> Demux/1
  Demux/1 -> Sum4/1  "chi_dot_ref"
  Kp/1 -> Sum4/2
  Sum4/1 -> Sum2/1
  Demux1/1 -> Discrete-Time Integrator/1, Kp/1
  Demux/2 -> Sum1/1  "gamma_dot_ref"
  CircleP1/1 -> Sum1/2
  Sum1/1 -> Sum3/1
  Demux1/2 -> Discrete-Time Integrator1/1, CircleP1/1
  Discrete-Time Integrator1/1 -> Gain5/1
  path_angles_a/1 -> Selector5/1, Selector3/1
  Sum/1 -> Mux1/2
  Selector4/1 -> Sum/1
  Selector2/1 -> wrapCourse/1(chi_ref)
  x_ref/1 -> Selector4/1, Selector2/1
  wrapCourse/1(e_course) -> Mux1/1
  Gain5/1 -> Gain/1
  Discrete-Time Integrator/1 -> Gain4/1
  Sum2/1 -> Mux/1
  Sum3/1 -> Mux/2
  Selector5/1 -> Sum/2
  Selector3/1 -> wrapCourse/2(chi)
  Gain/1 -> Sum3/2
  Gain4/1 -> Sum2/2

== system AWES3_CL_wTether_v4_PM/FlightController/Traction/FlightPathLoopTraction/EstimatePlantResponse ==
  mu_k_sat : Inport
  dphi : Inport  Port=2
  Ft : Inport  Port=3
  alpha_rq : Inport  Port=4
  chi_gamma_k : Inport  Port=5
  pos_O : Inport  Port=6
  v_k_B : Inport  Port=7
  airdata : Inport  Port=8
  Demux : Demux  Outputs=2
  MATLAB Function : MATLAB Function  TreatAsAtomicUnit=on
  Mux : Mux  Inputs=3
  Mux4 : Mux  Inputs=2
  Selector : Selector  InputPortWidth=3  IndexOptions=Index vector (dialog)  Indices=1  OutputSizes=1
  Selector1 : Selector  InputPortWidth=3  IndexOptions=Index vector (dialog)  Indices=3  OutputSizes=1
  pathAngleRate : Outport  VectorParamsAs1DForOutWhenUnconnected=off
  wires:
  MATLAB Function/2(gamma_dot_real) -> Mux4/2
  Mux4/1 -> pathAngleRate/1
  MATLAB Function/1(chi_dot_real) -> Mux4/1
  dphi/1 -> MATLAB Function/1(dphi)
  Demux/1 -> MATLAB Function/3(chi_k)
  Demux/2 -> MATLAB Function/4(gamma_k)
  Ft/1 -> MATLAB Function/5(F_t)
  mu_k_sat/1 -> MATLAB Function/2(mu_k)
  pos_O/1 -> MATLAB Function/6(pos_O)
  airdata/1 -> Selector1/1, Selector/1
  v_k_B/1 -> MATLAB Function/7(v_k_B)
  chi_gamma_k/1 -> Demux/1
  Selector/1 -> Mux/1
  Selector1/1 -> Mux/3
  alpha_rq/1 -> Mux/2
  Mux/1 -> MATLAB Function/8(airdata)

== system AWES3_CL_wTether_v4_PM/FlightController/Traction/Ft_set_smoothing/force switch1 ==
  u : Inport
  Delay : Delay  DelayLength=1
  Derivative : Derivative
  Gain : Gain  Gain=0.1
  MATLAB Function : MATLAB Function  TreatAsAtomicUnit=on
  Moving Average : dspstat3/Moving Average  Method=Sliding window  ForgettingFactorPort=off  SpecifyWindowLength=on  WindowLength=4  ForgettingFactor=0.9  SimulateUsing=Code generation
  Scope : Scope  NumInputPorts=4
  Subsystem : Subsystem
  sigma_new : Outport
  wires:
  Derivative/1 -> Gain/1
  Moving Average/1 -> Derivative/1
  u/1 -> Moving Average/1, Subsystem/1(Ft)  "force"
  Gain/1 -> Subsystem/2(dFt)  "predict force"
  Subsystem/1(mu_1) -> Scope/1, MATLAB Function/1(mu1)  "mu1"
  MATLAB Function/1(sigma) -> Delay/1, sigma_new/1
  Delay/1 -> MATLAB Function/5("sigma ")
  Subsystem/2(mu_2) -> Scope/2, MATLAB Function/2(mu2)
  Subsystem/3(mu_3) -> Scope/3, MATLAB Function/3(mu3)
  Subsystem/4(mu_4) -> Scope/4, MATLAB Function/4(mu4)

== system AWES3_CL_wTether_v4_PM/FlightController/Traction/Ft_set_smoothing/force switch2 ==
  u : Inport
  Clock : Clock
  Constant : Constant  Value=1500
  Constant1 : Constant  Value=Ft_max-30
  Constant2 : Constant  Value=Ft_max-50
  Constant3 : Constant  Value=0
  Delay : Delay  DelayLength=1  InitialCondition=0
  Derivative : Derivative
  Gain : Gain  Gain=0.1
  Gain1 : Gain  Gain=1/Ft_max
  Interval Test : simulink/Logic and Bit Operations/Interval Test  IntervalClosedRight=on  uplimit=inf  IntervalClosedLeft=on  lowlimit=1830  OutDataTypeStr=boolean
  Logical Operator : Logic  Operator=OR  IconShape=distinctive  AllPortsSameDT=off  OutDataTypeStr=boolean
  Logical Operator1 : Logic  IconShape=distinctive  AllPortsSameDT=off  OutDataTypeStr=boolean
  Logical Operator2 : Logic  Operator=OR  Inputs=3  IconShape=distinctive  AllPortsSameDT=off  OutDataTypeStr=boolean
  Moving Average : dspstat3/Moving Average  Method=Sliding window  ForgettingFactorPort=off  SpecifyWindowLength=on  WindowLength=4  ForgettingFactor=0.9  SimulateUsing=Code generation
  Relational Operator : RelationalOperator  Operator=<  OutDataTypeStr=boolean  RndMeth=Simplest  InputSameDT=off
  Relational Operator1 : RelationalOperator  Operator=<  OutDataTypeStr=boolean  RndMeth=Simplest  InputSameDT=off
  Relational Operator2 : RelationalOperator  Operator=<  OutDataTypeStr=boolean  RndMeth=Simplest  InputSameDT=off
  Scope : Scope  NumInputPorts=2
  Scope1 : Scope
  Sum : Sum  Inputs=|++
  Switch : Switch  Criteria=u2 > Threshold  Threshold=0.7  SaturateOnIntegerOverflow=off  InputSameDT=off
  Out : Outport
  wires:
  Constant1/1 -> Relational Operator/1
  Logical Operator2/1 -> Scope/1, Delay/1, Out/1
  Derivative/1 -> Gain/1
  Constant2/1 -> Relational Operator1/1
  Relational Operator1/1 -> Logical Operator2/3  "predict"
  Sum/1 -> Relational Operator1/2
  Interval Test/1 -> Logical Operator/1
  Constant3/1 -> Relational Operator2/1
  Gain1/1 -> Scope/2  "force"
  Logical Operator1/1 -> Logical Operator2/1  "hold"
  Delay/1 -> Logical Operator1/1
  Logical Operator/1 -> Logical Operator1/2
  Relational Operator/1 -> Logical Operator2/2  "exceed max"
  Gain/1 -> Sum/1, Scope1/1, Relational Operator2/2  "predict force"
  Moving Average/1 -> Derivative/1
  Relational Operator2/1 -> Logical Operator/2
  Constant/1 -> Switch/3
  u/1 -> Relational Operator/2, Interval Test/1, Switch/1, Sum/2, Moving Average/1  "force"
  Clock/1 -> Switch/2
  Switch/1 -> Gain1/1

== system AWES3_CL_wTether_v4_PM/FlightController/Traction/PI_controller_course/PI_controller_course_chi ==
  e_chi : Inport
  Kp : Gain  Gain=params.Kp_chi_k_traction  Multiplication=Matrix(K*u)
  Saturation1 : Saturate
  u_PI_fb : Outport  VectorParamsAs1DForOutWhenUnconnected=off
  wires:
  Kp/1 -> u_PI_fb/1  "nu_R"
  e_chi/1 -> Kp/1

== system AWES3_CL_wTether_v4_PM/FlightController/Traction/PI_controller_course/PI_controller_course_gamma ==
  e_gamma : Inport
  Kp : Gain  Gain=params.Kp_gamma_k_traction  Multiplication=Matrix(K*u)
  u_PI_fb : Outport  VectorParamsAs1DForOutWhenUnconnected=off
  wires:
  Kp/1 -> u_PI_fb/1  "nu_R"
  e_gamma/1 -> Kp/1

== system AWES3_CL_wTether_v4_PM/Aircraft_Winch_Tether/WinchDynamicsAndControl /PureTorqueControl/PI-ForceController/clamping_logic ==
  preSat : Inport
  preInt : Inport  Port=2
  control_def : Inport  Port=3
  AND3 : Logic  DisableCoverage=on  OutDataTypeStr=boolean
  Constant1 : Constant  DisableCoverage=on  Value=0  OutDataTypeStr=Inherit: Inherit via back propagation  PreserveConstantTs=on
  DataTypeConv1 : DataTypeConversion  DisableCoverage=on  OutDataTypeStr=int8  SaturateOnIntegerOverflow=off  RndMeth=Floor
  DataTypeConv2 : DataTypeConversion  DisableCoverage=on  OutDataTypeStr=int8  SaturateOnIntegerOverflow=off  RndMeth=Floor
  Equal1 : RelationalOperator  DisableCoverage=on  Operator===  OutDataTypeStr=boolean  RndMeth=Floor  InputSameDT=off
  Memory : Memory  DisableCoverage=on  InheritSampleTime=on
  NotEqual : RelationalOperator  DisableCoverage=on  Operator=~=  OutDataTypeStr=boolean  RndMeth=Floor  InputSameDT=off
  SignPreIntegrator : Signum  DisableCoverage=on
  SignPreSat : Signum  DisableCoverage=on
  Switch : Switch  Criteria=u2 > Threshold  SaturateOnIntegerOverflow=off
  ZeroGain : Gain  DisableCoverage=on  Gain=0  OutDataTypeStr=Inherit: Same as input  ParamDataTypeStr=Inherit: Same as input
  deadzone around zero : DeadZone  LowerValue=-1e-9  UpperValue=1e-9
  pre_integration_processed : Outport  VectorParamsAs1DForOutWhenUnconnected=off
  wires:
  AND3/1 -> Memory/1
  Equal1/1 -> AND3/2
  deadzone around zero/1 -> NotEqual/2, SignPreSat/1
  Memory/1 -> Switch/2
  control_def/1 -> deadzone around zero/1
  Constant1/1 -> Switch/1
  DataTypeConv1/1 -> Equal1/1
  DataTypeConv2/1 -> Equal1/2
  SignPreSat/1 -> DataTypeConv1/1
  preInt/1 -> SignPreIntegrator/1, Switch/3
  NotEqual/1 -> AND3/1
  SignPreIntegrator/1 -> DataTypeConv2/1
  ZeroGain/1 -> NotEqual/1
  preSat/1 -> ZeroGain/1
  Switch/1 -> pre_integration_processed/1
